simulink model "BD_PAR_AUTO_base_model"  (Simulink 10.3)
settings: Solver=ode1  StartTime=0.0  StopTime=max(cyc_mph(:,1))  FixedStep=1  MaxStep=1  RelTol=1e-3  AbsTol=1e-3
undefined symbols (not defined in the file): acc_dcdc_eff, acc_elec_eff, acc_elec_pwr, acc_mech_eff, acc_mech_pwr, acc_mech_trq, air_cp, amb_tmp, cs_charge_deplete_bool, cs_charge_trq, cs_electric_decel_spd, cs_electric_launch_spd_hi, cs_electric_launch_spd_lo, cs_hi_soc, cs_lo_soc, cs_min_trq_frac, cs_off_trq_frac, cyc_avg_time, cyc_cargo_mass, cyc_elevation_init, cyc_filter_bool, cyc_grade, cyc_mph, enable_sim_stop_distance, enable_sim_stop_max_spd, enable_sim_stop_speed, enable_sim_stop_time, enable_stop, enable_stop_fc, ess_cap_scale, ess_coulombic_eff, ess_init_soc, ess_max_ah_cap, ess_max_volts, ess_min_volts, ess_mod_airflow, ess_mod_cp, ess_mod_init_tmp, ess_module_mass, ess_module_num, ess_on, ess_r_chg, ess_r_dis, ess_res_scale_coef, ess_res_scale_fun, ess_set_tmp, ess_soc, ess_th_calc, ess_th_res_off, ess_th_res_on, ess_tmp, ess_voc, ex_calc, ex_cat_co_frac, ex_cat_ext_cp, ex_cat_ext_emisv, ex_cat_ext_init_tmp, ex_cat_ext_mass, ex_cat_ext_sarea, ex_cat_hc_frac ... (+168)
(part 1 of 15)
settings Model: Creator=mokeefe  LastModifiedBy=thyag  ExtModeTrigMode=oneshot  ExtModeArmWhenConnect=off
settings Model: ModifiedComment=|
  | mokeefe -- Fri Apr 06 09:23:46 2012 -- Version 1.22
  | Restore all library links and save to latest version.
settings Model: ModifiedHistory=|
  | mokeefe -- Fri Apr 06 09:23:46 2012 -- Version 1.22
  | Restore all library links and save to latest version.
  | 
  | mokeefe -- Fri Apr 06 09:23:46 2012 -- Version 1.22
  | Restore all library links and save to latest version.
  | 
  | ssprik -- Wed Sep 24 15:05:16 2003 -- Version 1.21
  | 
  | 
  | mokeefe -- Fri Aug 30 07:45:49 2002 -- Version 1.20
  | Changed the input to "mechanical accessory loads <acc>/Mechanical Accessory Loads V2 <acc>" masked parameter input blocks. In R13, the function "not" no longer returns double 1 or double 0 for true and false but instead returns type logical (boolean). Thus, I am now multiplying by double 1 which causes a type conversion to double yielding the desired effect.
  | 
  | 
  | abrooker -- Tue May 14 11:45:21 2002 -- Version 1.19
  | 
  | 
  | mokeefe -- Thu Apr 18 08:00:10 2002 -- Version 1.18
  | saving the model:
  | o "without the model browser open"
  | o with only top-level screen visible
  | o and with "fit to view" enabled
settings SolverCC: AutoScaleAbsTol=off
settings DataIOCC: SaveOutput=off  SaveTime=off
settings OptimizationCC: BooleanDataType=off
settings DebuggingCC: SaveWithParameterizedLinksMsg=none  SignalResolutionControl=TryResolveAllWithWarning  MultiTaskDSMMsg=warning  MultiTaskCondExecSysMsg=none  UnconnectedLineMsg=none
settings HardwareCC: TargetUnknown=on
settings RTWCC: TemplateMakefile=grt_vc.tmf

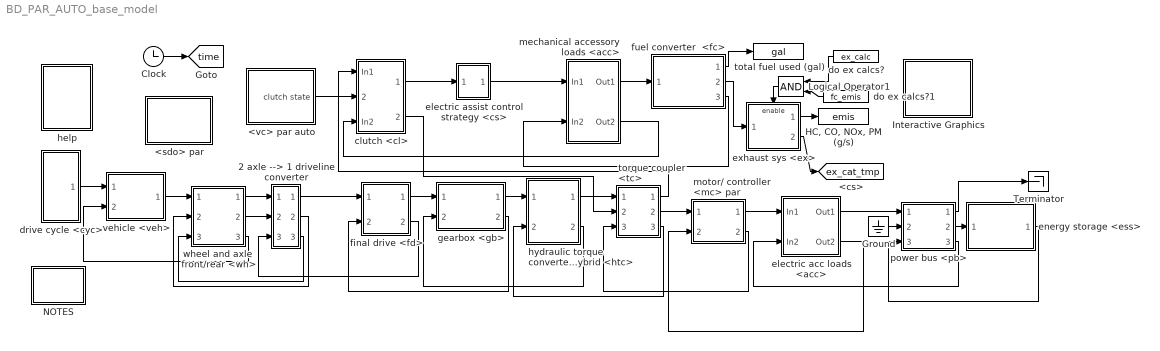
== system BD_PAR_AUTO_base_model ==
  2 axle --> 1 driveline converter : Subsystem
  <sdo> par : Subsystem
      mask Display: image(imread('bdi_sdo.jpg'))
  <vc> par auto : Subsystem
      mask Display: image(imread('bdi_vc.jpg'))
  Clock : Clock
  Ground : Ground
  "HC, CO, NOx, PM (g/s)" : ToWorkspace  VariableName=emis
  Interactive Graphics : Subsystem  BlockChoice=off
      settings: AttributesFormatString=%<BlockChoice>  TemplateBlock=lib_interactive/Interactive Graphics  MemberBlocks=off,on
  Logical Operator1 : Logic
  NOTES : Subsystem
      mask Display: disp('Version &\nCopyright')
  Terminator : Terminator
  clutch <cl> : Subsystem  mask(Clutch){slip_spd=vc_launch_spd, maxtrq=max(fc_max_trq)*fc_trq_scale}
      mask prompts: slip_spd "Input shaft speed when clutch slips (rad/s):"; maxtrq "Maximum torque clutch can transmit:"
      mask help: Clutch for use with ADVISOR 2
      mask Help:
      | First input is req'd clutch output torque and speed, muxed together.
      | Second input is clutch state, with 1 => disengaged, 2 => slipping, and 3=> engaged.
      | Third input is available clutch input torque and limited clutch input speed.
      | First output is req'd clutch input torque and speed, muxed together.
      | Second output is available clutch output torque and limited clutch output speed.
      | The logic implemented by this block is as follows:
      |           IF (clutch is disengaged) THEN (req'd input torque=0), (req'd input speed=req'd output speed (the engine control is responsible for computing correct engine spin-down speed)), (avail. output torque=0), (limited output speed=req'd output speed)
      |           IF (clutch is slipping) THEN (req'd input torque=req'd output torque), (req'd input speed=user-defined slip speed), (avail. output torque=avail. input torque), (limited output speed=req'd output speed)
      |           IF (clutch is engaged) THEN (req'd input torque=req'd output torque), (req'd input speed=req'd output speed), (avail. output torque=avail. input torque), (limited output speed=limited input speed)
      | 
      | The clutch will transmit no more than its maximum torque as driving or braking torque.
      mask Display: image(imread('bdi_cl.jpg'))
  do ex calcs? : Constant  Value=ex_calc
  do ex calcs?1 : Constant  Value=fc_emis
  drive cycle <cyc> : Subsystem
      mask Display: image(imread('bdi_cyc.jpg'))
  electric acc loads <acc> : Subsystem
      mask Display: image(imread('bdi_acc_elec.bmp'))
  electric assist control strategy <cs> : Subsystem
      mask Display: image(imread('bdi_cs.jpg'))
  energy storage <ess> : Subsystem
      mask Display: image(imread('bdi_ess.jpg'))
  exhaust sys <ex> : Subsystem  TreatAsAtomicUnit=on
      mask Display: image(imread('bdi_ex.jpg'))
  final drive <fd> : Subsystem
      mask Display: image(imread('bdi_fd.jpg'))
  fuel converter  <fc> : Subsystem
      mask Display: image(imread('bdi_fc.jpg'))
  gearbox <gb> : Subsystem
      mask Display: image(imread('bdi_gb.jpg'))
  help : Subsystem
      settings: OpenFcn=web(['file:\\\' which('advisor_doc.htm')]);
      mask Display: image(imread('doc_man.jpg'))
  hydraulic torque converter for  parallel hybrid <htc> : Subsystem
      mask Display: image(imread('bdi_htc.jpg'))
  mechanical accessory loads <acc> : Subsystem
      mask Display: image(imread('bdi_acc_pic.bmp'))
  motor/ controller <mc> par : Subsystem
      mask Display: image(imread('bdi_mc.jpg'))
  power bus <pb> : Subsystem
      mask Display: image(imread('bdi_pb.jpg'))
  torque coupler <tc> : Subsystem
      mask Display: image(imread('bdi_tc.jpg'))
  total fuel used (gal) : ToWorkspace  VariableName=gal
  vehicle <veh> : Subsystem
      mask Display: image(imread('bdi_veh.jpg'))
  wheel and axle  front/rear <wh> : Subsystem
      mask Display: image(imread('bdi_wh.jpg'))
  tag scope: ex_cat_tmp=global, time=global
  wires:
  vehicle <veh>/1("tractive force and speed required of tire and wheel (N), (m/s)") -> wheel and axle  front/rear <wh>/1("tractive force and speed req'd of tire/road interface (N), (m/s)")
  wheel and axle  front/rear <wh>/3(tractive force and linear speed  achievable) -> vehicle <veh>/2(tractive force and linear speed achievable (N))
  2 axle --> 1 driveline converter/1(req) -> final drive <fd>/1("torque and speed req'd at output side of final drive (Nm), (rad/s)")
  final drive <fd>/2("torque and speed avail. at output side of final drive (Nm), (rad/s)") -> 2 axle --> 1 driveline converter/3(ach)
  final drive <fd>/1("torque and speed req'd at input side of final drive (Nm), (rad/s)") -> gearbox <gb>/1("torque and speed req'd at output side of gearbox (Nm), (rad/s)")
  drive cycle <cyc>/1(req'd vehicle speed (m/s)) -> vehicle <veh>/1(vehicle speed req'd at end of time step (m/s))
  clutch <cl>/1(Out1) -> electric assist control strategy <cs>/1("trq and spd req'd into clutch (N*m, rad/s)")
  fuel converter  <fc>/2(EO emis info) -> exhaust sys <ex>/1(EO emis info)
  do ex calcs?/1 -> Logical Operator1/1
  fuel converter  <fc>/1(fuel use) -> total fuel used (gal)/1
  exhaust sys <ex>/1(tailpipe emis (g/s)) -> "HC, CO, NOx, PM (g/s)"/1
  Logical Operator1/1 -> exhaust sys <ex>/Enable
  do ex calcs?1/1 -> Logical Operator1/2
  Clock/1 -> [time]
  gearbox <gb>/2("torque and speed avail. at output side of gearbox (Nm), (rad/s)") -> final drive <fd>/2("torque and speed avail. at input side of final drive (Nm), (rad/s)")
  clutch <cl>/2(Out2) -> torque coupler <tc>/2("torque and speed avail. at main input (Nm), (rad/s)")
  <vc> par auto/1(clutch state) -> clutch <cl>/2(clutch state: 1 => disengaged 2 => slipping 3 => engaged)
  torque coupler <tc>/1("torque and speed req'd at main input to torque coupler (Nm), (rad/s)") -> clutch <cl>/1(In1)
  motor/ controller <mc> par/2("drive torque and speed avail. at rotor (Nm), (rad/s)") -> torque coupler <tc>/3("torque and speed avail. at motor input to tc (Nm), (rad/s)")
  Ground/1 -> power bus <pb>/2(power available from generator (W))
  power bus <pb>/2(power req'd from energy storage (W)) -> energy storage <ess>/1(power req'd into bus (W))
  power bus <pb>/1(power req'd from generator (W)) -> Terminator/1
  energy storage <ess>/1(power available to bus (W)) -> power bus <pb>/3(power available from energy storage (W))
  torque coupler <tc>/2("torque and speed req'd at motor input to torque coupler (Nm), (rad/s)") -> motor/ controller <mc> par/1("torque and speed  req'd at rotor (Nm), (rad/s)")
  gearbox <gb>/1("torque and speed req'd at input side of gearbox (Nm), (rad/s)") -> hydraulic torque converter for  parallel hybrid <htc>/1("req'd output trq and spd (Nm), (rad/s)")
  hydraulic torque converter for  parallel hybrid <htc>/1("req'd input trq and spd (Nm), (rad/s)") -> torque coupler <tc>/1("torque and speed req'd at output side of torque coupler (Nm), (rad/s)")
  hydraulic torque converter for  parallel hybrid <htc>/2("trq and spd available at output (Nm), (rad/s)") -> gearbox <gb>/2("torque and speed avail. at input side of gearbox (Nm), (rad/s)")
  torque coupler <tc>/3("torque and speed avail. at output side of torque coupler (Nm), (rad/s)") -> hydraulic torque converter for  parallel hybrid <htc>/2("trq and spd available at input (Nm), (rad/s)")
  exhaust sys <ex>/2(cat tmp (C)) -> [ex_cat_tmp]
  motor/ controller <mc> par/1(req'd motor input power (W)) -> electric acc loads <acc>/1(In1)
  electric acc loads <acc>/1(Out1) -> power bus <pb>/1(req'd power output (W))
  power bus <pb>/3(output power  available at bus) -> electric acc loads <acc>/2(In2)
  electric acc loads <acc>/2(Out2) -> motor/ controller <mc> par/2(available motor input power (W))
  electric assist control strategy <cs>/1("trq and spd req'd from engine (N*m, rad/s)") -> mechanical accessory loads <acc>/1(In1)
  mechanical accessory loads <acc>/1(Out1) -> fuel converter  <fc>/1(torque and speed  req'd at engine  output shaft (Nm))
  fuel converter  <fc>/3("torque and speed  avail. to driveline (Nm), (rad/s)") -> mechanical accessory loads <acc>/2(In2)
  mechanical accessory loads <acc>/2(Out2) -> clutch <cl>/3(In2)
  wheel and axle  front/rear <wh>/1(torque and speed req'd from drivetrain into front axle (Nm),(rad/s)) -> 2 axle --> 1 driveline converter/1(front req)
  wheel and axle  front/rear <wh>/2(torque and speed req'd from drivetrain into rear axle (Nm),(rad/s)) -> 2 axle --> 1 driveline converter/2(rear req)
  2 axle --> 1 driveline converter/2(front ach) -> wheel and axle  front/rear <wh>/2("torque and speed available from drivetrain into front axle (Nm), (rad/s)")
  2 axle --> 1 driveline converter/3(rear ach) -> wheel and axle  front/rear <wh>/3("torque and speed available from drivetrain into rear axle (Nm), (rad/s)")

== system BD_PAR_AUTO_base_model/2 axle --> 1 driveline converter ==
  front req : Inport
  rear req : Inport  Port=2
  ach : Inport  Port=3
  Constant : Constant  Value=wh_front_active_bool
  Constant1 : Constant  Value=wh_rear_active_bool
  Constant2 : Constant  Value=wh_front_active_bool
  Constant3 : Constant  Value=wh_rear_active_bool
  Constant4 : Constant  Value=eps
  Constant5 : Constant  Value=0
  Demux : Demux  Outputs=2
  Demux1 : Demux  Outputs=2
  Demux2 : Demux  Outputs=2
  Ground : Ground
  Logical Operator : Logic  Operator=NAND
  Mux{,1..3} (4 alike) : Mux  Inputs=2
  Product : Product  Inputs=*/  SaturateOnIntegerOverflow=on
  Product1 : Product  SaturateOnIntegerOverflow=on
  Sum : Sum  SaturateOnIntegerOverflow=on
  Sum1 : Sum  Inputs=+-  SaturateOnIntegerOverflow=on
  Sum2 : Sum  SaturateOnIntegerOverflow=on
  Switch{,1..6} (7 alike) : Switch  Threshold=eps
  Terminator : Terminator
  req : Outport
  front ach : Outport  Port=2
  rear ach : Outport  Port=3
  wires:
  Constant5/1 -> Switch6/3
  Switch6/1 -> Sum1/2, Mux2/1
  Product1/1 -> Switch6/1
  Sum2/1 -> Product/2
  Constant4/1 -> Sum2/2
  Demux2/2 -> Mux3/2, Mux2/2, Mux1/2
  Switch5/1 -> Switch4/1
  Switch2/1 -> Switch3/1
  Mux1/1 -> Switch5/3
  Mux2/1 -> Switch2/3
  Mux3/1 -> Switch3/3, Switch4/3
  Ground/1 -> Mux3/1
  Constant2/1 -> Switch3/2
  Constant3/1 -> Switch4/2
  Sum1/1 -> Mux1/1
  Product/1 -> Product1/1
  Demux2/1 -> Sum1/1, Product1/2
  Switch4/1 -> rear ach/1
  Switch3/1 -> front ach/1
  ach/1 -> Switch5/1, Switch2/1, Demux2/1
  Constant1/1 -> Logical Operator/2
  front req/1 -> Switch/1, Demux/1
  Demux1/2 -> Terminator/1
  Demux/2 -> Mux/2
  Sum/1 -> Switch6/2, Sum2/1, Mux/1
  Demux/1 -> Product/1, Sum/1
  Demux1/1 -> Sum/2
  Mux/1 -> Switch1/3
  Switch1/1 -> req/1
  Logical Operator/1 -> Switch5/2, Switch2/2, Switch1/2
  Switch/1 -> Switch1/1
  Constant/1 -> Logical Operator/1, Switch/2
  rear req/1 -> Switch/3, Demux1/1

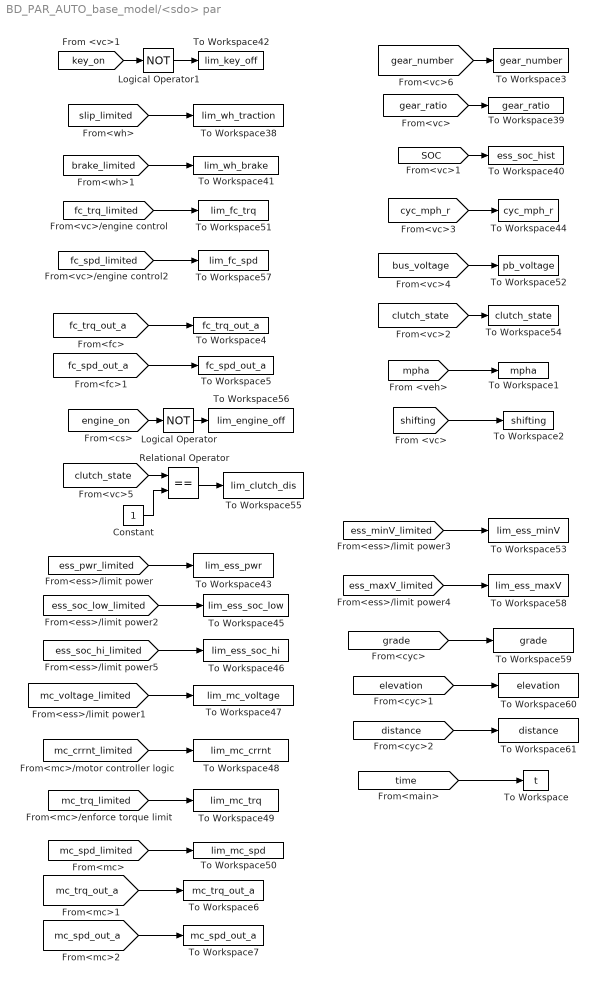
== system BD_PAR_AUTO_base_model/<sdo> par ==
  Constant : Constant
  Logical Operator : Logic  Operator=NOT  Inputs=1
  Logical Operator1 : Logic  Operator=NOT  Inputs=1
  Relational Operator : RelationalOperator  Operator===  RndMeth=Nearest  InputSameDT=on
  To Workspace : ToWorkspace  VariableName=t
  To Workspace1 : ToWorkspace  VariableName=mpha  SampleTime=-1
  To Workspace2 : ToWorkspace  VariableName=shifting  SampleTime=-1
  To Workspace3 : ToWorkspace  VariableName=gear_number  SampleTime=-1
  To Workspace38 : ToWorkspace  VariableName=lim_wh_traction  SampleTime=-1
  To Workspace39 : ToWorkspace  VariableName=gear_ratio  SampleTime=-1
  To Workspace4 : ToWorkspace  VariableName=fc_trq_out_a  SampleTime=-1
  To Workspace40 : ToWorkspace  VariableName=ess_soc_hist  SampleTime=-1
  To Workspace41 : ToWorkspace  VariableName=lim_wh_brake  SampleTime=-1
  To Workspace42 : ToWorkspace  VariableName=lim_key_off  SampleTime=-1
  To Workspace43 : ToWorkspace  VariableName=lim_ess_pwr  SampleTime=-1
  To Workspace44 : ToWorkspace  VariableName=cyc_mph_r  SampleTime=-1
  To Workspace45 : ToWorkspace  VariableName=lim_ess_soc_low  SampleTime=-1
  To Workspace46 : ToWorkspace  VariableName=lim_ess_soc_hi  SampleTime=-1
  To Workspace47 : ToWorkspace  VariableName=lim_mc_voltage  SampleTime=-1
  To Workspace48 : ToWorkspace  VariableName=lim_mc_crrnt  SampleTime=-1
  To Workspace49 : ToWorkspace  VariableName=lim_mc_trq  SampleTime=-1
  To Workspace5 : ToWorkspace  VariableName=fc_spd_out_a  SampleTime=-1
  To Workspace50 : ToWorkspace  VariableName=lim_mc_spd  SampleTime=-1
  To Workspace51 : ToWorkspace  VariableName=lim_fc_trq  SampleTime=-1
  To Workspace52 : ToWorkspace  VariableName=pb_voltage  SampleTime=-1
  To Workspace53 : ToWorkspace  VariableName=lim_ess_minV  SampleTime=-1
  To Workspace54 : ToWorkspace  VariableName=clutch_state  SampleTime=-1
  To Workspace55 : ToWorkspace  VariableName=lim_clutch_dis  SampleTime=-1
  To Workspace56 : ToWorkspace  VariableName=lim_engine_off  SampleTime=-1
  To Workspace57 : ToWorkspace  VariableName=lim_fc_spd  SampleTime=-1
  To Workspace58 : ToWorkspace  VariableName=lim_ess_maxV  SampleTime=-1
  To Workspace59 : ToWorkspace  VariableName=grade  SampleTime=-1
  To Workspace6 : ToWorkspace  VariableName=mc_trq_out_a  SampleTime=-1
  To Workspace60 : ToWorkspace  VariableName=elevation  SampleTime=-1
  To Workspace61 : ToWorkspace  VariableName=distance  SampleTime=-1
  To Workspace7 : ToWorkspace  VariableName=mc_spd_out_a  SampleTime=-1
  wires:
  [gear_number] -> To Workspace3/1
  [mc_spd_out_a] -> To Workspace7/1
  [mc_trq_out_a] -> To Workspace6/1
  [time] -> To Workspace/1
  [fc_spd_out_a] -> To Workspace5/1
  [fc_trq_out_a] -> To Workspace4/1
  Relational Operator/1 -> To Workspace55/1
  [mc_spd_limited] -> To Workspace50/1
  [mc_trq_limited] -> To Workspace49/1
  [mc_crrnt_limited] -> To Workspace48/1
  [mc_voltage_limited] -> To Workspace47/1
  [ess_soc_hi_limited] -> To Workspace46/1
  [ess_soc_low_limited] -> To Workspace45/1
  Logical Operator/1 -> To Workspace56/1
  [engine_on] -> Logical Operator/1
  Constant/1 -> Relational Operator/2
  [clutch_state] -> Relational Operator/1
  [ess_pwr_limited] -> To Workspace43/1
  [distance] -> To Workspace61/1
  [elevation] -> To Workspace60/1
  [grade] -> To Workspace59/1
  [ess_minV_limited] -> To Workspace53/1
  [ess_maxV_limited] -> To Workspace58/1
  [brake_limited] -> To Workspace41/1
  [slip_limited] -> To Workspace38/1
  Logical Operator1/1 -> To Workspace42/1
  [key_on] -> Logical Operator1/1
  [shifting] -> To Workspace2/1
  [mpha] -> To Workspace1/1
  [clutch_state] -> To Workspace54/1
  [bus_voltage] -> To Workspace52/1
  [SOC] -> To Workspace40/1
  [cyc_mph_r] -> To Workspace44/1
  [gear_ratio] -> To Workspace39/1
  [fc_spd_limited] -> To Workspace57/1
  [fc_trq_limited] -> To Workspace51/1

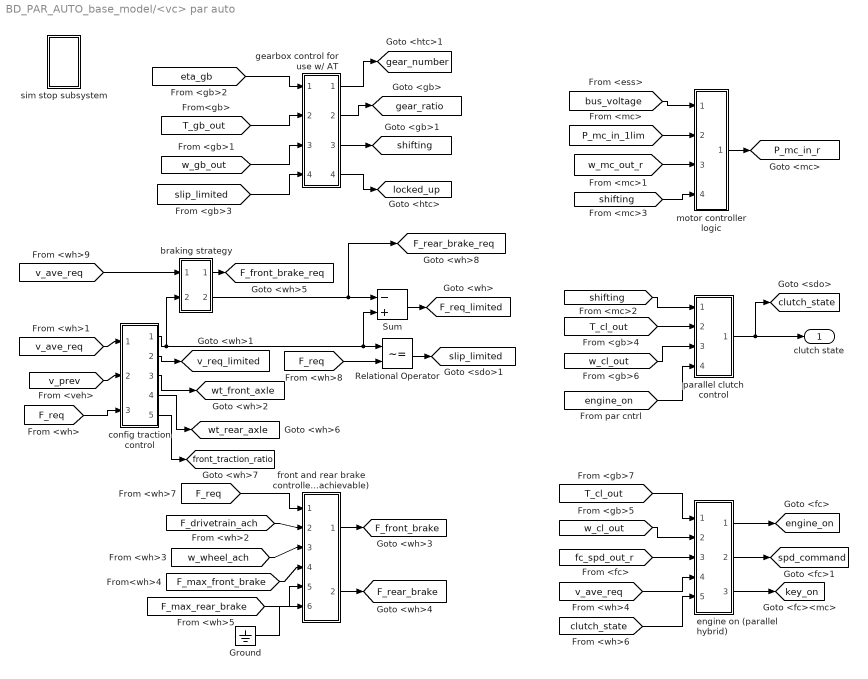
== system BD_PAR_AUTO_base_model/<vc> par auto ==
  Ground : Ground
  Relational Operator : RelationalOperator  Operator=~=  RndMeth=Nearest  InputSameDT=on
  Sum : Sum  Inputs=-+  InputSameDT=on  SaturateOnIntegerOverflow=on  OutDataTypeStr=Inherit: Same as first input
  braking strategy : Subsystem
  config traction control : Subsystem  BlockChoice=traction control 2 axle
      settings: AttributesFormatString=%<BlockChoice>  TemplateBlock=lib_controls/SubSystem/config traction control  MemberBlocks=traction control 2 axle,traction control J2452 2 axle
  engine on (parallel hybrid) : Subsystem
  front and rear brake controller (achievable) : Subsystem
  gearbox control for use w/ AT : Subsystem
  motor controller logic : Subsystem
  parallel clutch control : Subsystem
  sim stop subsystem : Subsystem
  clutch state : Outport
  tag scope: F_front_brake=global, F_front_brake_req=global, F_rear_brake=global, F_rear_brake_req=global, F_req_limited=global, P_mc_in_r=global, clutch_state=global, engine_on=global, front_traction_ratio=global, gear_number=global, gear_ratio=global, key_on=global, locked_up=global, shifting=global, slip_limited=global, spd_command=global, v_req_limited=global, wt_front_axle=global, wt_rear_axle=global
  wires:
  Ground/1 -> front and rear brake controller (achievable)/6(tractive force available from  rear drivetrain (N))
  config traction control/5(front/total  traction ratio) -> [front_traction_ratio]
  config traction control/4(weight on rear axle (N)) -> [wt_rear_axle]
  gearbox control for use w/ AT/3("shifting, out") -> [shifting]
  gearbox control for use w/ AT/2("gear ratio, out") -> [gear_ratio]
  gearbox control for use w/ AT/1("gear number, out") -> [gear_number]
  [engine_on] -> parallel clutch control/4(engine on)
  [T_cl_out] -> parallel clutch control/2(gb_trq_in_r)
  [w_cl_out] -> parallel clutch control/3(gb_spd_in_r)
  [shifting] -> parallel clutch control/1(shifting)
  parallel clutch control/1(clutch state) -> clutch state/1, [clutch_state]
  [clutch_state] -> engine on (parallel hybrid)/5(clutch state)
  [v_ave_req] -> engine on (parallel hybrid)/4(v_ave_req)
  engine on (parallel hybrid)/1(engine on) -> [engine_on]
  [T_cl_out] -> engine on (parallel hybrid)/1(trq req'd out of clutch (N*m))
  [w_cl_out] -> engine on (parallel hybrid)/2(spd req'd out of clutch (N*m)1)
  engine on (parallel hybrid)/3(key on) -> [key_on]
  [fc_spd_out_r] -> engine on (parallel hybrid)/3(fc_spd_out_r)
  engine on (parallel hybrid)/2(spd command  (rad/s)) -> [spd_command]
  [F_req] -> Relational Operator/2
  Relational Operator/1 -> [slip_limited]
  Sum/1 -> [F_req_limited]
  braking strategy/2(req'd rear brake force (N)) -> [F_rear_brake_req], Sum/1
  [F_req] -> front and rear brake controller (achievable)/1(total tractive force req'd (N))
  front and rear brake controller (achievable)/1(front-axle braking force (N)) -> [F_front_brake]
  [F_drivetrain_ach] -> front and rear brake controller (achievable)/2(tractive force available from  front drivetrain (N))
  [w_wheel_ach] -> front and rear brake controller (achievable)/3(axle speed possible (rad/s))
  [F_max_front_brake] -> front and rear brake controller (achievable)/4(max front brake force (N))
  [F_max_rear_brake] -> front and rear brake controller (achievable)/5(max rear brake force (N))
  front and rear brake controller (achievable)/2(rear-axle braking force (N)) -> [F_rear_brake]
  [v_ave_req] -> braking strategy/1(req'd speed (m/s))
  [v_ave_req] -> config traction control/1(time-average vehicle speed  req'd (m/s))
  [F_req] -> config traction control/3(total tractive force req'd (N))
  config traction control/1(req'd force (N)) -> Relational Operator/1, Sum/2, braking strategy/2(slip-limited force req'd (N))
  braking strategy/1(req'd front brake force (N)) -> [F_front_brake_req]
  [v_prev] -> config traction control/2(vehicle speed at beginning of time  step (m/s))
  config traction control/2(req'd speed (m/s)) -> [v_req_limited]
  config traction control/3(weight on front axle (N)) -> [wt_front_axle]
  gearbox control for use w/ AT/4(locked up) -> [locked_up]
  [slip_limited] -> gearbox control for use w/ AT/4(tires are at traction limit)
  [w_gb_out] -> gearbox control for use w/ AT/3(gb_spd_out_r)
  [T_gb_out] -> gearbox control for use w/ AT/2(gb_trq_out_r)
  [eta_gb] -> gearbox control for use w/ AT/1(eta_gb)
  [shifting] -> motor controller logic/4(shifting)
  [bus_voltage] -> motor controller logic/1(bus voltage)
  [P_mc_in_1lim] -> motor controller logic/2(req'd input power (W))
  [w_mc_out_r] -> motor controller logic/3(req'd output spd (rad/s))
  motor controller logic/1(req'd input power (W)1) -> [P_mc_in_r]

== system BD_PAR_AUTO_base_model/Interactive Graphics ==
  off : Subsystem  Tag=Altia_off
      mask Display: image(imread('results.bmp'))

== system BD_PAR_AUTO_base_model/NOTES ==
  note: ADVISOR software developed at NREL.  Copyright 1998 Midwest Research Institute.  All rights reserved.
      | Notice: These data were produced by the Midwest Research Institute (MRI) under Contract No. DE-AC98GO10337
      |      with the Department of Energy (DOE).  For a five-year period from November 6, 1998, the Government is granted for
      | itself and others acting on its behalf a nonexclusive, paid-up, irrevocable worldwide license in this data to reproduce,
      |  prepare derivative works, and perform publicly and display publicly, by or on behalf of the Government.  There is
      | provision for the possible extension of the term of this license.  Subsequent to that period or any extension granted,
      |  the Government is granted for itself and others acting on its behalf a nonexclusive, paid-up, irrevocable worldwide
  note: license in this data to reproduce, prepare derivative works, distribute copies to the public, perform publicly and display
      | publicly, and to permit others to do so.  The specific term of the license can be identified by inquiry made to the MRI
      | or DOE. Neither the United States nor the DOE, nor any of their employees, make any warranty, express or implied, or
      | assumes any legal liability or responsibility for the accuracy, completeness, or usefulness of any data, apparatus,
      | product, or process disclosed, or represents that its use would not infringe privately owned rights.
  NOTES : Subsystem
      settings: OpenFcn=advisor_ver
      mask Display: disp('Double-click here or enter ''advisor_ver'' at the Matlab\ncommand line for ADVISOR version')

== system BD_PAR_AUTO_base_model/clutch <cl> ==
  In1 : Inport
  clutch state: 1 => disengaged 2 => slipping 3 => engaged : Inport  Port=2
  In2 : Inport  Port=3
  Constant : Constant
  Constant1 : Constant  Value=2
  Constant2 : Constant  Value=3
  Constant3 : Constant  Value=0
  Constant4 : Constant  Value=slip_spd
  Constant5 : Constant  Value=0
  Demux : Demux  Outputs=2
  Demux1 : Demux  Outputs=2
  Logical Operator : Logic  Operator=NOT  Inputs=1
  Logical Operator1 : Logic  Operator=NOT  Inputs=1
  Logical Operator2 : Logic  Operator=NOT  Inputs=1
  Mux : Mux  Inputs=2
  Mux1 : Mux  Inputs=2
  Product : Product  Inputs=1  SaturateOnIntegerOverflow=on
  Product1 : Product  Inputs=1  SaturateOnIntegerOverflow=on
  Saturation : Saturate  UpperLimit=maxtrq  LowerLimit=-maxtrq
  Saturation1 : Saturate  UpperLimit=maxtrq  LowerLimit=-maxtrq
  Switch{,1..3} (4 alike) : Switch  Threshold=eps
  To Workspace1 : ToWorkspace  VariableName=clutch_pwr_in_a  SampleTime=-1
  To Workspace2 : ToWorkspace  VariableName=clutch_pwr_out_a  SampleTime=-1
  clutch disengaged : RelationalOperator  Operator===  RndMeth=Nearest  InputSameDT=on
  clutch engaged : RelationalOperator  Operator===  RndMeth=Nearest  InputSameDT=on
  clutch slipping : RelationalOperator  Operator===  RndMeth=Nearest  InputSameDT=on
  help : Subsystem
      settings: OpenFcn=web(['file:\\\' which('clutch.htm')]);
      mask Display: image(imread('doc_man.jpg'))
  Out1 : Outport
  Out2 : Outport  Port=2
  tag scope: T_cl_out=global, w_cl_out=global
  wires:
  Mux1/1 -> Product1/1, Out2/1
  Product1/1 -> To Workspace2/1
  Product/1 -> To Workspace1/1
  In2/1 -> Product/1, Demux1/1
  Demux/2 -> [w_cl_out], Switch3/3, Switch1/1  "output speed req'd"
  Demux/1 -> [T_cl_out], Switch/1  "output torque"
  clutch engaged/1 -> Switch3/2
  Switch3/1 -> Mux1/2
  Demux1/2 -> Switch3/1
  Constant5/1 -> Switch2/3
  Logical Operator2/1 -> Switch2/2
  Demux1/1 -> Switch2/1
  Switch1/1 -> Mux/2
  Constant4/1 -> Switch1/3
  Logical Operator1/1 -> Switch1/2
  Constant3/1 -> Switch/3
  Logical Operator/1 -> Switch/2
  clutch disengaged/1 -> Logical Operator2/1, Logical Operator/1  "clutch disengaged"
  clutch slipping/1 -> Logical Operator1/1
  Constant2/1 -> clutch engaged/2
  Mux/1 -> Out1/1
  In1/1 -> Demux/1
  clutch state: 1 => disengaged 2 => slipping 3 => engaged/1 -> clutch engaged/1, clutch slipping/1, clutch disengaged/1
  Constant1/1 -> clutch slipping/2
  Constant/1 -> clutch disengaged/2
  Switch2/1 -> Saturation/1
  Saturation/1 -> Mux1/1
  Switch/1 -> Saturation1/1
  Saturation1/1 -> Mux/1

== system BD_PAR_AUTO_base_model/drive cycle <cyc> ==
  Backlash : Backlash  BacklashWidth=0.5
  Block NOTES : Subsystem
      mask Display: disp('Block\nNOTES')
  Constant : Constant  Value=0.001
  Constant1 : Constant  Value=0
  Constant2 : Constant  Value=cyc_filter_bool
  Derivative : Derivative
  Integrator : Integrator  InitialCondition=cyc_elevation_init
  Product : Product  InputSameDT=on  RndMeth=Zero  SaturateOnIntegerOverflow=on  OutDataTypeStr=Inherit: Same as first input
  Relational Operator : RelationalOperator  Operator=>  RndMeth=Nearest  InputSameDT=on
  Switch : Switch  Threshold=eps
  Switch1 : Switch  Threshold=eps
  Switch2 : Switch  Threshold=1
  Switch3 : Switch  Threshold=1
  To Workspace : ToWorkspace  VariableName=veh_cargo_mass_vs_time  SampleTime=-1
  To Workspace1 : ToWorkspace  VariableName=ambient_pressure  SampleTime=-1
  Trigonometric Function : Trigonometry
  ambient pressure calc (atm) : Subsystem
  distance travelled (m) : Subsystem
  mph-->m/s : Gain  Gain=0.447  SaturateOnIntegerOverflow=on  OutDataTypeStr=Inherit: Same as input  ParamDataTypeStr=Inherit: Same as input
  repeated cycle grade vs. distance : Subsystem  mask(Repeating table){t=cyc_grade(:,1), y=cyc_grade(:,2)}
      mask prompts: t "Input values:"; y "Output values:"
      mask help:
      | Repeating table.
      | Enter values of input and output for first cycle.
      mask init:
      | period = max(t);
      mask Help: Repeats cycle given in table. Input values should be monotonically increasing.
  repeated cycle speed vs. time : Subsystem  mask(Repeating table){t=cyc_mph(:,1), y=cyc_mph(:,2)}
      mask prompts: t "Time values:"; y "Output values:"
      mask help:
      | Repeating table.
      | Enter values of time and output for first cycle.
      mask init:
      | period = max(t);
      mask Help: Repeats cycle given in table. Time values should be monotonically increasing.
  repeated cycle vehicle cargo mass vs. distance : Subsystem  mask(Repeating table){t=cyc_cargo_mass(:,1), y=cyc_cargo_mass(:,2)}
      mask prompts: t "Input values:"; y "Output values:"
      mask help:
      | Repeating table.
      | Enter values of input and output for first cycle.
      mask init:
      | period = max(t);
      mask Help: Repeats cycle given in table. Input values should be monotonically increasing.
  "super-smooth, no-lag trace" : Subsystem  mask(Smooth Cycle){t=cyc_mph(:,1), y=cyc_mph(:,2), avgtime=cyc_avg_time}
      mask prompts: t "Time vector for trace (s):"; y "Speed vector for trace (km/hr):"; avgtime "Averaging time (s):"
      mask help: Smooth Cycle
      mask init:
      | period = max(t);,
      mask Display: disp('SMOOTH\nCYCLE')
  req'd vehicle speed (m/s) : Outport  InitialOutput=0
  tag scope: cyc_mph_r=global, cyc_mph_r_orig=global, distance=global, elevation=global, grade=global, grade_orig=global, veh_cargo_mass=global
  wires:
  [elevation] -> ambient pressure calc (atm)/1(elevation)
  ambient pressure calc (atm)/1(Out1) -> To Workspace1/1
  repeated cycle vehicle cargo mass vs. distance/1(out_1) -> To Workspace/1, [veh_cargo_mass]
  [Altia_Run] -> Switch3/2
  [altia_grade] -> Switch3/1
  [Altia_Run] -> Switch2/2
  [altia_cyc_mph_r] -> Switch2/1
  mph-->m/s/1 -> req'd vehicle speed (m/s)/1
  Switch2/1 -> mph-->m/s/1, [cyc_mph_r]
  Constant2/1 -> Switch1/2
  Constant1/1 -> Switch/3
  Relational Operator/1 -> Switch/2
  Backlash/1 -> Switch/1
  Constant/1 -> Relational Operator/2
  "super-smooth, no-lag trace"/1(out_1) -> Relational Operator/1, Backlash/1
  Switch/1 -> Switch1/1
  repeated cycle speed vs. time/1(out_1) -> Switch1/3
  Switch1/1 -> [cyc_mph_r_orig], Switch2/3
  Product/1 -> Integrator/1
  Derivative/1 -> Product/1
  Trigonometric Function/1 -> Product/2
  Integrator/1 -> [elevation]
  Switch3/1 -> [grade], Trigonometric Function/1
  distance travelled (m)/1(Out1) -> repeated cycle vehicle cargo mass vs. distance/1(distance travelled (m)), [distance], Derivative/1, repeated cycle grade vs. distance/1(distance travelled (m))
  repeated cycle grade vs. distance/1(out_1) -> Switch3/3, [grade_orig]

== system BD_PAR_AUTO_base_model/electric acc loads <acc> ==
  note: from vc
  In1 : Inport
  In2 : Inport  Port=2
  Electrical Accessory Loads v2 <acc> : Subsystem  mask{load_on=ess_on}
      mask prompts: load_on "1 to enable loads; 0 to disable"
      mask Display: image(imread('bdi_acc_elec.bmp'))
  Out1 : Outport
  Out2 : Outport  Port=2
  wires:
  In1/1 -> Electrical Accessory Loads v2 <acc>/1("requested electrical Power, out to the driveline (W)")
  In2/1 -> Electrical Accessory Loads v2 <acc>/2(achieved power in from power source (W))
  Electrical Accessory Loads v2 <acc>/1("requested electrical Power, in from the power source (W)") -> Out1/1
  Electrical Accessory Loads v2 <acc>/2("achieved electrical Power, out to the driveline (W)") -> Out2/1
  [key_on] -> Electrical Accessory Loads v2 <acc>/3(on/off)

== system BD_PAR_AUTO_base_model/electric assist control strategy <cs> ==
  "trq and spd req'd into clutch (N*m, rad/s)" : Inport
  Constant : Constant  Value=0
  Demux : Demux  Outputs=2
      settings: DisplayOption=none
  MinMax : MinMax  Function=max  Inputs=2  InputSameDT=on  SaturateOnIntegerOverflow=on
  Mux : Mux  Inputs=2
  Sum : Sum  InputSameDT=on  SaturateOnIntegerOverflow=on  OutDataTypeStr=Inherit: Same as first input
  Switch : Switch  Threshold=eps
  chg trq req'd (Nm) : Subsystem
  help : Subsystem
      settings: OpenFcn=web(['file:\\\' which('Parallel.htm')])
      mask Display: image(imread('doc_man.jpg'))
  minimum trq (Nm) : Subsystem
  "trq and spd req'd from engine (N*m, rad/s)" : Outport
  wires:
  Demux/1 -> Sum/2
  [engine_on] -> Switch/2
  minimum trq (Nm)/1(minimum trq (N*m)) -> MinMax/2
  Demux/2 -> Mux/2
  Mux/1 -> "trq and spd req'd from engine (N*m, rad/s)"/1
  Switch/1 -> Mux/1
  Constant/1 -> Switch/3
  MinMax/1 -> Switch/1
  Sum/1 -> MinMax/1
  chg trq req'd (Nm)/1(add'l trq req'd (Nm)) -> Sum/1
  "trq and spd req'd into clutch (N*m, rad/s)"/1 -> Demux/1, minimum trq (Nm)/1("trq and spd req'd into trq coupler (N*m, rad/s)")

== system BD_PAR_AUTO_base_model/energy storage <ess> ==
  power req'd into bus (W) : Inport
  ess config : Subsystem  BlockChoice=energy storage <ess>
      settings: AttributesFormatString=%<BlockChoice>  TemplateBlock=lib_energy_storage/Ess Choices/ess config  MemberBlocks="Ultracapacitor  System,energy storage <ess>,energy storage <ess> RC,energy storage <ess> nnet,energy storage <ess> Saber,energy storage <ess> fundamental model,energy storage <ess> optima fundamental model"
  power available to bus (W) : Outport  InitialOutput=0
  wires:
  power req'd into bus (W)/1 -> ess config/1(power req'd into bus (W))
  ess config/1(power available to bus (W)) -> power available to bus (W)/1

== system BD_PAR_AUTO_base_model/exhaust sys <ex> ==
  note: EO emis
  note: fc on?
  EO emis info : Inport
  Enable : EnablePort  StatesWhenEnabling=reset
  1-u : MATLABFcn  MATLABFcn=1.0-u
  1/Ccm : Gain  Gain=1/(ex_cat_mon_mass*fc_pwr_scale*ex_cat_mon_cp)  SaturateOnIntegerOverflow=on
  1/Ccp : Gain  Gain=1/(ex_cat_pipe_mass*fc_pwr_scale*ex_cat_pipe_cp)  SaturateOnIntegerOverflow=on
  1/Ccx : Gain  Gain=1/(ex_cat_ext_mass*fc_pwr_scale*ex_cat_ext_cp)  SaturateOnIntegerOverflow=on
  1/Cm : Gain  Gain=1/(ex_manif_mass*fc_pwr_scale*ex_manif_cp)  SaturateOnIntegerOverflow=on
  Block NOTES : Subsystem
      mask Display: disp('Block\nNOTES')
  Break- thru : MATLABFcn  MATLABFcn=u-ex_cat_lim
  Demux1 : Demux  Outputs=[1 4 1 1 1 1 4]
  Demux2 : Demux
  MinMax : MinMax  Function=max  Inputs=2
  Mux1 : Mux  Inputs=2
  Mux3 : Mux  Inputs=5
  PCM : Lookup  InputValues=ex_cat_pcm_tmp  Table=ex_cat_pcm_ecp
  Q/Cci : Fcn  Expr=u(2)/(ex_cat_int_mass*fc_pwr_scale*ex_cat_int_cp+ex_cat_pcm_mass*u(1))
  Qci : Sum  Inputs=-+  SaturateOnIntegerOverflow=on
  Qcm : Sum  Inputs=+-+  SaturateOnIntegerOverflow=on
  Qcp : Sum  Inputs=-+  SaturateOnIntegerOverflow=on
  Qcp3 : Sum  Inputs=+-  SaturateOnIntegerOverflow=on
  Qm : Sum  Inputs=-+  SaturateOnIntegerOverflow=on
  Saturation3 : Saturate  UpperLimit=Inf  LowerLimit=0
  Saturation4 : Saturate  UpperLimit=Inf  LowerLimit=eps
  Tci : Integrator  InitialCondition=ex_cat_int_init_tmp
  Tcm : Integrator  InitialCondition=ex_cat_mon_init_tmp
  Tcp : Integrator  InitialCondition=ex_cat_pipe_init_tmp
  Tcx : Integrator  InitialCondition=ex_cat_ext_init_tmp
  Tm : Integrator  InitialCondition=ex_manif_init_tmp
  To Workspace10 : ToWorkspace  VariableName=ex_cat_tmp  SampleTime=-1
  To Workspace11 : ToWorkspace  VariableName=ex_tmp  SampleTime=-1
  To Workspace14 : ToWorkspace  VariableName=ex_cat_th_pwr  SampleTime=-1
  To Workspace15 : ToWorkspace  VariableName=ex_cat_eff  SampleTime=-1
  To Workspace8 : ToWorkspace  VariableName=ex_gas_tmp  SampleTime=-1
  ex gas heat flow : Subsystem  TreatAsAtomicUnit=on
  ex sys heat flow : Subsystem
  help : Subsystem
      settings: OpenFcn=web(['file:\\\' which('exhaust.htm')]);
      mask Display: image(imread('doc_man.jpg'))
  removal efficiencies : Subsystem
  tailpipe  emis : Product  SaturateOnIntegerOverflow=on
  tot cat eff1 : Product  Inputs=/*  SaturateOnIntegerOverflow=on
  tailpipe emis (g/s) : Outport  OutputWhenDisabled=reset  InitialOutput=0
  cat tmp (C) : Outport  Port=2  OutputWhenDisabled=reset  InitialOutput=0
  wires:
  Demux1/5 -> removal efficiencies/3(O2_exh (g/s))
  Demux1/7 -> ex sys heat flow/2(Tfc,x)
  Demux1/6 -> ex sys heat flow/1(veh spd)
  Demux1/2 -> removal efficiencies/4(emis Engine Out (g/s)), Qcp3/1, Break- thru/1, tailpipe  emis/1, Saturation4/1
  Demux1/3 -> removal efficiencies/1(gas_flow (g/s)), ex gas heat flow/2(ex gas flow)
  ex gas heat flow/1(Tex,gas) -> removal efficiencies/2(Ex Gas T (C)), To Workspace8/1
  EO emis info/1 -> Demux1/1
  tot cat eff1/1 -> To Workspace15/1
  Saturation4/1 -> tot cat eff1/1
  Saturation3/1 -> tot cat eff1/2, ex gas heat flow/1(emis cat'd)
  Qcp3/1 -> Saturation3/1
  removal efficiencies/1(removal effs) -> 1-u/1
  MinMax/1 -> Qcp3/2, tailpipe emis (g/s)/1
  1-u/1 -> tailpipe  emis/2
  tailpipe  emis/1 -> MinMax/2
  Break- thru/1 -> MinMax/1
  ex gas heat flow/2(Qcat) -> To Workspace14/1, Qcm/1
  1/Ccp/1 -> Tcp/1
  Qcp/1 -> 1/Ccp/1
  Tcm/1 -> To Workspace10/1, removal efficiencies/5(Ex Cat T (C)), cat tmp (C)/1, Mux3/1
  Mux3/1 -> ex sys heat flow/3(ex_temp), ex gas heat flow/4(ex_temp), To Workspace11/1
  Tm/1 -> Mux3/5
  Tcp/1 -> Mux3/3
  Tcx/1 -> Mux3/4
  Demux2/3 -> Qcp/1
  Demux2/4 -> Qm/1
  Demux2/2 -> Qci/1
  ex sys heat flow/3(Qcat_p) -> Qcp/2
  Tci/1 -> Mux3/2, PCM/1
  Qci/1 -> Mux1/2
  PCM/1 -> Mux1/1
  Mux1/1 -> Q/Cci/1
  Q/Cci/1 -> Tci/1
  Qm/1 -> 1/Cm/1
  1/Cm/1 -> Tm/1
  1/Ccx/1 -> Tcx/1
  ex sys heat flow/2(Qcat_i) -> Qci/2
  ex sys heat flow/5(Qmanif) -> Qm/2
  ex sys heat flow/4(Qcat_x) -> 1/Ccx/1
  Demux2/1 -> Qcm/2
  ex sys heat flow/1(Qcat_m) -> Qcm/3
  Qcm/1 -> 1/Ccm/1
  1/Ccm/1 -> Tcm/1
  Demux1/1 -> ex gas heat flow/Enable
  Demux1/4 -> ex gas heat flow/3(Tex,eo)
  ex gas heat flow/3(Qex) -> Demux2/1

== system BD_PAR_AUTO_base_model/final drive <fd> ==
  "torque and speed req'd at output side of final drive (Nm), (rad/s)" : Inport
  "torque and speed avail. at input side of final drive (Nm), (rad/s)" : Inport  Port=2
  Block NOTES : Subsystem
      mask Display: disp('Block\nNOTES')
  Demux : Demux  Outputs=2
  Demux1 : Demux  Outputs=2
  Gain : Gain  Gain=fd_ratio  SaturateOnIntegerOverflow=on
  Gain1 : Gain  Gain=1/fd_ratio  SaturateOnIntegerOverflow=on
  Gain2 : Gain  Gain=fd_ratio  SaturateOnIntegerOverflow=on
  Gain3 : Gain  Gain=1/fd_ratio  SaturateOnIntegerOverflow=on
  Mux : Mux  Inputs=2
  Mux1 : Mux  Inputs=2
  Sum1 : Sum  Inputs=--+  SaturateOnIntegerOverflow=on
  Sum2 : Sum  Inputs=+++  SaturateOnIntegerOverflow=on
  To Workspace2 : ToWorkspace  VariableName=fd_trq_out_r  SampleTime=-1
  To Workspace3 : ToWorkspace  VariableName=fd_spd_out_r  SampleTime=-1
  To Workspace4 : ToWorkspace  VariableName=fd_trq_in_r  SampleTime=-1
  To Workspace5 : ToWorkspace  VariableName=fd_spd_in_r  SampleTime=-1
  To Workspace6 : ToWorkspace  VariableName=fd_trq_in_a  SampleTime=-1
  To Workspace7 : ToWorkspace  VariableName=fd_spd_in_a  SampleTime=-1
  To Workspace8 : ToWorkspace  VariableName=fd_trq_out_a  SampleTime=-1
  To Workspace9 : ToWorkspace  VariableName=fd_spd_out_a  SampleTime=-1
  effect of inertia (Nm) : Subsystem
  help : Subsystem
      settings: OpenFcn=web(['file:\\\' which('wheel_axle.htm')]);
      mask Display: image(imread('doc_man.jpg'))
  loss (Nm) : Subsystem
  "torque and speed req'd at input side of final drive (Nm), (rad/s)" : Outport  InitialOutput=0
  "torque and speed avail. at output side of final drive (Nm), (rad/s)" : Outport  Port=2  InitialOutput=0
  wires:
  Gain2/1 -> To Workspace8/1, Mux1/1
  Gain3/1 -> To Workspace9/1, Mux1/2
  Demux1/2 -> To Workspace7/1, Gain3/1
  Demux1/1 -> To Workspace6/1, Sum1/3
  Sum2/1 -> To Workspace4/1, Mux/1
  Demux/2 -> To Workspace3/1, Gain/1
  Demux/1 -> To Workspace2/1, Gain1/1
  Mux/1 -> "torque and speed req'd at input side of final drive (Nm), (rad/s)"/1
  "torque and speed req'd at output side of final drive (Nm), (rad/s)"/1 -> Demux/1
  Gain1/1 -> Sum2/1
  Gain/1 -> To Workspace5/1, Mux/2, effect of inertia (Nm)/1(fd input speed (rad/s)), loss (Nm)/1(fd output speed (rad/s))
  effect of inertia (Nm)/1(drag torque (Nm)) -> Sum2/3, Sum1/2
  loss (Nm)/1(drag torque (Nm)) -> Sum2/2, Sum1/1
  Mux1/1 -> "torque and speed avail. at output side of final drive (Nm), (rad/s)"/1
  "torque and speed avail. at input side of final drive (Nm), (rad/s)"/1 -> Demux1/1
  Sum1/1 -> Gain2/1

== system BD_PAR_AUTO_base_model/fuel converter  <fc> ==
  torque and speed  req'd at engine  output shaft (Nm) : Inport
  Block NOTES : Subsystem
      mask Display: disp('Block\nNOTES')
  Demux : Demux  Outputs=2
      settings: DisplayOption=none
  Mux : Mux  Inputs=2
  Mux1 : Mux  Inputs=2
  To Workspace2 : ToWorkspace  VariableName=fc_trq_out_r  SampleTime=-1
  To Workspace3 : ToWorkspace  VariableName=fc_spd_out_r  SampleTime=-1
  To Workspace7 : ToWorkspace  VariableName=fc_brake_trq  SampleTime=-1
  To Workspace9 : ToWorkspace  VariableName=fc_spd_est  SampleTime=-1
  engine controller interface : Subsystem
  engine speed estimator : Subsystem
  engine torque : Subsystem
  fuel use and EO emis Configurable Subsystem : Subsystem  BlockChoice=fuel use and EO emis
      settings: AttributesFormatString=%<BlockChoice>  TemplateBlock=lib_fuel_converter/configurable subsystems/fuel use and EO emis Configurable Subsystem  MemberBlocks=fuel use and EO emis,fuel use and EO emis Neural Network Model
  help : Subsystem
      settings: OpenFcn=web(['file:\\\' which('fuel_converter.htm')]);
      mask Display: image(imread('doc_man.jpg'))
  fuel use : Outport  InitialOutput=0
  EO emis info : Outport  Port=2  InitialOutput=0
  "torque and speed  avail. to driveline (Nm), (rad/s)" : Outport  Port=3  InitialOutput=0
  tag scope: fc_brake_trq=global, fc_spd_est=global, fc_spd_out_a=global, fc_trq_out_a=global, fuel=global
  wires:
  engine speed estimator/1(Out1) -> [fc_spd_est], To Workspace9/1, fuel use and EO emis Configurable Subsystem/2(w (rad/s)), engine torque/3(engine spd)
  fuel use and EO emis Configurable Subsystem/1(cumulative fuel  use (gal)) -> [fuel], fuel use/1
  Demux/2 -> [fc_spd_out_r], To Workspace3/1, engine controller interface/1(fc_spd_out_r)
  torque and speed  req'd at engine  output shaft (Nm)/1 -> Demux/1
  Demux/1 -> To Workspace2/1, engine torque/1(fc_trq_out_r)
  engine controller interface/1(spd command) -> Mux1/2, [fc_spd_out_a], engine speed estimator/1(spd command), engine torque/2(spd command)
  Mux/1 -> EO emis info/1
  fuel use and EO emis Configurable Subsystem/2("FC ON?, EOem, MFex, Tex, O2ex") -> Mux/1
  fuel use and EO emis Configurable Subsystem/3(Vv,Tfc) -> Mux/2
  Mux1/1 -> "torque and speed  avail. to driveline (Nm), (rad/s)"/1
  engine torque/1(map torque (Nm)) -> [fc_brake_trq], To Workspace7/1, fuel use and EO emis Configurable Subsystem/1(T (Nm))
  engine torque/2(torque to shaft (Nm)) -> Mux1/1, [fc_trq_out_a]

== system BD_PAR_AUTO_base_model/gearbox <gb> ==
  "torque and speed req'd at output side of gearbox (Nm), (rad/s)" : Inport
  "torque and speed avail. at input side of gearbox (Nm), (rad/s)" : Inport  Port=2
  Block NOTES : Subsystem
      mask Display: disp('Block\nNOTES')
  Constant : Constant  Value=0
  Demux : Demux  Outputs=2
  Demux1 : Demux  Outputs=2
  Logical Operator : Logic  Operator=NOT  Inputs=1
  Memory : Memory
  Mux : Mux  Inputs=2
  Mux1 : Mux  Inputs=2
  "Pout/Pin, neglecting inertia" : Subsystem
  Product : Product  SaturateOnIntegerOverflow=on
  Product1 : Product  SaturateOnIntegerOverflow=on
  Sum2 : Sum  Inputs=+++  SaturateOnIntegerOverflow=on
  Sum3 : Sum  Inputs=-+  SaturateOnIntegerOverflow=on
  Switch : Switch  Threshold=eps
  To Workspace10 : ToWorkspace  VariableName=gb_ni_trq_out_a  SampleTime=-1
  To Workspace2 : ToWorkspace  VariableName=gb_trq_out_r  SampleTime=-1
  To Workspace3 : ToWorkspace  VariableName=gb_spd_out_r  SampleTime=-1
  To Workspace4 : ToWorkspace  VariableName=gb_trq_out_a  SampleTime=-1
  To Workspace5 : ToWorkspace  VariableName=gb_spd_out_a  SampleTime=-1
  To Workspace6 : ToWorkspace  VariableName=gb_trq_in_a  SampleTime=-1
  To Workspace7 : ToWorkspace  VariableName=gb_spd_in_a  SampleTime=-1
  To Workspace8 : ToWorkspace  VariableName=gb_trq_in_r  SampleTime=-1
  To Workspace9 : ToWorkspace  VariableName=gb_spd_in_r  SampleTime=-1
  effect of inertia (Nm) : Subsystem
  gearbox controller interface : Subsystem
  "gearing (Nm), (rad/s)" : Subsystem
  "gearing (Nm), (rad/s)1" : Subsystem
  help : Subsystem
      settings: OpenFcn=web(['file:\\\' which('gearbox.htm')]);
      mask Display: image(imread('doc_man.jpg'))
  loss (Nm) : Subsystem  mask{tx_eff_map=tx_eff_map, tx_map_trq=tx_map_trq, tx_map_spd=tx_map_spd, gb_spd_scale=gb_spd_scale, gb_trq_scale=gb_trq_scale}
      mask prompts: tx_eff_map "table of efficiency values (spd rad/s, trq Nm)"; tx_map_trq "vector of output torque values for lookup table (Nm)"; tx_map_spd "vector of output speeds for lookup table (rad/s)"; gb_spd_scale "Speed scale for the transmission gear box"; gb_trq_scale "Torque scale for the transmission gear box"
  "torque and speed req'd at input side of gearbox (Nm), (rad/s)" : Outport  InitialOutput=0
  "torque and speed avail. at output side of gearbox (Nm), (rad/s)" : Outport  Port=2  InitialOutput=0
  tag scope: gb_spd_in_a=global
  wires:
  [gear_number] -> loss (Nm)/3(gear_number)
  Product1/1 -> To Workspace10/1
  Product/1 -> Product1/2, Sum3/2
  Mux1/1 -> "torque and speed avail. at output side of gearbox (Nm), (rad/s)"/1
  Sum3/1 -> "gearing (Nm), (rad/s)1"/1(input shaft torque (Nm))
  "torque and speed avail. at input side of gearbox (Nm), (rad/s)"/1 -> Demux1/1
  "Pout/Pin, neglecting inertia"/1(Pout/Pin) -> Memory/1, Product/1
  Memory/1 -> gearbox controller interface/3(eta_gb)
  Mux/1 -> "torque and speed req'd at input side of gearbox (Nm), (rad/s)"/1
  "gearing (Nm), (rad/s)"/1(input shaft torque (Nm)) -> Sum2/1
  "gearing (Nm), (rad/s)"/2(input shaft speed (rad/s)) -> effect of inertia (Nm)/1(gb input speed (rad/s)), Mux/2, To Workspace9/1
  effect of inertia (Nm)/1(drag torque (Nm)) -> Sum2/3, Sum3/1, "Pout/Pin, neglecting inertia"/2(Tinertia)
  "torque and speed req'd at output side of gearbox (Nm), (rad/s)"/1 -> "gearing (Nm), (rad/s)"/1("output shaft torque and speed  (Nm), (rad/s)"), loss (Nm)/1("output torque and speed (Nm), (rad/s)"), Demux/1
  Demux/2 -> gearbox controller interface/2(w_gb_out), To Workspace3/1
  Demux/1 -> gearbox controller interface/1(T_gb_out), "Pout/Pin, neglecting inertia"/3(Tout), To Workspace2/1
  "gearing (Nm), (rad/s)1"/2(output shaft speed (rad/s)) -> Mux1/2, To Workspace5/1
  "gearing (Nm), (rad/s)1"/1(output shaft torque (Nm)) -> Mux1/1, To Workspace4/1
  Demux1/1 -> Product/2, To Workspace6/1
  Demux1/2 -> "gearing (Nm), (rad/s)1"/2(input shaft speed (rad/s)), To Workspace7/1, [gb_spd_in_a]
  Sum2/1 -> "Pout/Pin, neglecting inertia"/1(Tin), Switch/1
  gearbox controller interface/2(shifting) -> Logical Operator/1
  Logical Operator/1 -> Switch/2
  Switch/1 -> To Workspace8/1, Mux/1
  Constant/1 -> Switch/3
  loss (Nm)/1(loss torque at input shaft (Nm)) -> Sum2/2
  gearbox controller interface/1(gear_ratio) -> loss (Nm)/2(gear ratio), "gearing (Nm), (rad/s)"/2(gear ratio), Product1/1, "gearing (Nm), (rad/s)1"/3(gear ratio), "Pout/Pin, neglecting inertia"/4(gear ratio)

== system BD_PAR_AUTO_base_model/help ==
